simulink model "model_example"  (R2018b)
settings: Solver=FixedStepAuto  StartTime=0.0  StopTime=Tsim  FixedStep=Ts  RelTol=1e-3
undefined symbols (not defined in the file): a, b, c, x0
settings Model: Creator=palmisanom  LastModifiedBy=palmisanom

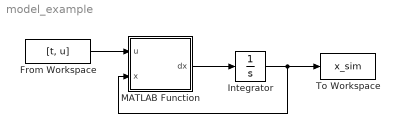
== system model_example ==
  From Workspace : FromWorkspace  VariableName=[t, u]  SampleTime=0
  Integrator : Integrator  InitialCondition=x0
  MATLAB Function : MATLAB Function  TreatAsAtomicUnit=on
  To Workspace : ToWorkspace  VariableName=x_sim  SaveFormat=Structure With Time  SampleTime=-1
  wires:
  MATLAB Function/1(dx) -> Integrator/1
  Integrator/1 -> To Workspace/1, MATLAB Function/2(x)
  From Workspace/1 -> MATLAB Function/1(u)

== matlab function model_example/MATLAB Function ==
  data: u input; dx output; x input; a parameter; b parameter; c parameter
function dx = fcn(u,x,a,b,c)
dx = [0;0];

dx(1) = x(2);
dx(2) = 1/a * (b*cos(x(1)) + c*u);
